simulink model "WiFiPDRFuzzyLogic20201103"  (R2016b)
settings: Solver=FixedStepDiscrete  StartTime=0.0  StopTime=260  FixedStep=1  RelTol=1e-3
libraries: fuzblock x1, simulink x1
settings Model: Creator=yyk  LastModifiedBy=yan_k
settings SolverCC: ZeroCrossAlgorithm=Adaptive

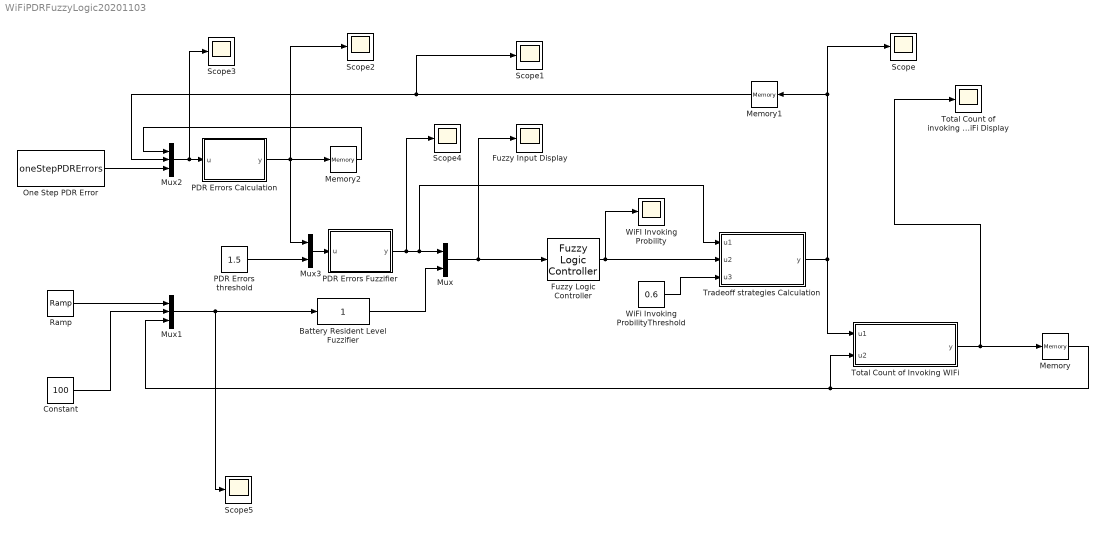
== system WiFiPDRFuzzyLogic20201103 ==
  Battery Resident Level Fuzzifier : Fcn  Expr=1
  Constant : Constant  Value=100
  Fuzzy Input Display : Scope
  Fuzzy Logic Controller : fuzblock/Fuzzy Logic  Controller  fis=wifipdrfuzzy2
  Memory : Memory
  Memory1 : Memory
  Memory2 : Memory
  Mux : Mux  Inputs=2
  Mux1 : Mux  Inputs=3
  Mux2 : Mux  Inputs=[1 1 1]
  Mux3 : Mux  Inputs=2
  One Step PDR Error : FromWorkspace  VariableName=oneStepPDRErrors  SampleTime=0
  PDR Errors Calculation : MATLAB Function  TreatAsAtomicUnit=on
  PDR Errors Fuzzifier : MATLAB Function  TreatAsAtomicUnit=on
  "PDR Errors threshold " : Constant  Value=1.5
  Ramp : simulink/Sources/Ramp  slope=1  start=0  X0=0
  Scope{,1..5} (6 alike) : Scope
  Total Count of Invoking WIFi : MATLAB Function  TreatAsAtomicUnit=on
  Total Count of invoking WiFi Display : Scope
  Tradeoff strategies Calculation : MATLAB Function  TreatAsAtomicUnit=on
  WiFI Invoking Probility : Scope
  "WiFi Invoking ProbilityThreshold " : Constant  Value=0.6
  wires:
  Mux/1 -> Fuzzy Input Display/1, Fuzzy Logic Controller/1
  Battery Resident Level Fuzzifier/1 -> Mux/2
  Mux1/1 -> Scope5/1, Battery Resident Level Fuzzifier/1
  Constant/1 -> Mux1/2
  Mux2/1 -> Scope3/1, PDR Errors Calculation/1(u)
  Fuzzy Logic Controller/1 -> Tradeoff strategies Calculation/2(u2), WiFI Invoking Probility/1
  "WiFi Invoking ProbilityThreshold "/1 -> Tradeoff strategies Calculation/3(u3)
  Tradeoff strategies Calculation/1(y) -> Total Count of Invoking WIFi/1(u1), Scope/1, Memory1/1
  Memory/1 -> Mux1/3, Total Count of Invoking WIFi/2(u2)
  Total Count of Invoking WIFi/1(y) -> Memory/1, Total Count of invoking WiFi Display/1
  Memory1/1 -> Scope1/1, Mux2/2
  Ramp/1 -> Mux1/1
  PDR Errors Calculation/1(y) -> Memory2/1, Scope2/1, Mux3/1
  Memory2/1 -> Mux2/1
  PDR Errors Fuzzifier/1(y) -> Scope4/1, Tradeoff strategies Calculation/1(u1), Mux/1
  "PDR Errors threshold "/1 -> Mux3/2
  Mux3/1 -> PDR Errors Fuzzifier/1(u)
  One Step PDR Error/1 -> Mux2/3

== matlab function WiFiPDRFuzzyLogic20201103/PDR Errors Calculation ==
  data: u input; y output

function y = fcn(u)

        resetSignal=u(2);
        oneStepError=u(3);
       
        if resetSignal ==1 
            lastSumPDRErrors = 0;
        else 
            lastSumPDRErrors = u(1);
        end 
        errors = lastSumPDRErrors + oneStepError
        y=errors
        
  end

== matlab function WiFiPDRFuzzyLogic20201103/Tradeoff strategies Calculation ==
  data: u1 input; y output; u2 input; u3 input
function y = fcn(u1,u2,u3)
     wifiProbThrod = u3
     wifiProb = u2
     
    if (wifiProb >=wifiProbThrod || u1==1  )
        y = 1;
    else
        y=0;
    end
end

== matlab function WiFiPDRFuzzyLogic20201103/Total Count of Invoking WIFi ==
  data: u1 input; y output; u2 input
function y = fcn(u1,u2)
y = u1+u2;

== matlab function WiFiPDRFuzzyLogic20201103/PDR Errors Fuzzifier ==
  data: u input; y output
function y = fcn(u)
    maxPDRErrors = u(2)
    if u(1) < maxPDRErrors
        y= u(1)/maxPDRErrors;
    else u(1) >= maxPDRErrors
        y =1;
    end
end
